simulink model "Cau_7_TDM_PCM"  (R2019a)
settings: Solver=VariableStepAuto  StartTime=0.0  StopTime=10.0  RelTol=1e-3
libraries: commutil2 x4, dspquant2 x4, dsparch4 x2, dspsigops x2, dspindex x1
settings Model: Creator=Thanh_Hai  LastModifiedBy=Thanh_Hai

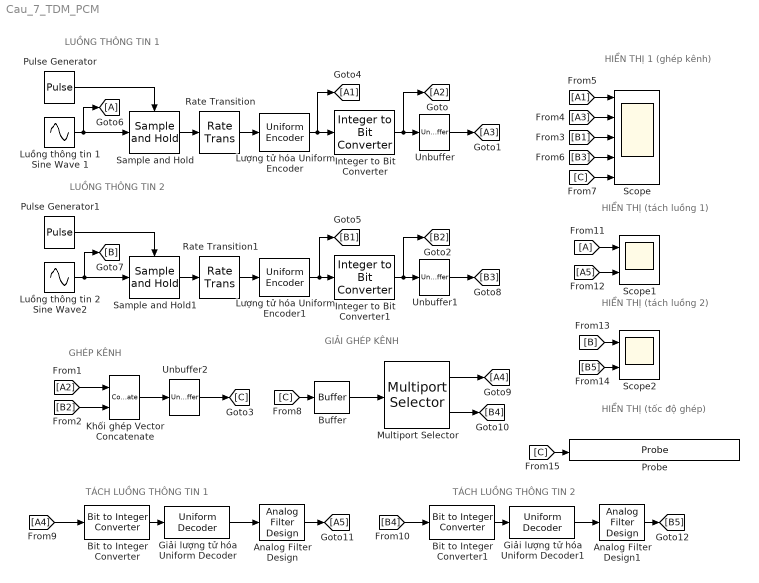
== system Cau_7_TDM_PCM ==
  note: GHÉP KÊNH
  note: LUỒNG THÔNG TIN 2
  note: HIỂN THỊ 1
      | (ghép kênh)
  note: LUỒNG THÔNG TIN 1
  note: HIỂN THỊ
      | (tách luồng 2)
  note: HIỂN THỊ
      | (tách luồng 1)
  note: GIẢI GHÉP KÊNH
  note: TÁCH LUỒNG THÔNG TIN 1
  note: TÁCH LUỒNG THÔNG TIN 2
  note: HIỂN THỊ
      | (tốc độ ghép)
  Analog Filter Design : dsparch4/Analog Filter Design  method=Butterworth  filttype=Lowpass  N=12  Wlo=2*pi*2500  Whi=80  Rp=2  Rs=40
  Analog Filter Design1 : dsparch4/Analog Filter Design  method=Butterworth  filttype=Lowpass  N=12  Wlo=2*pi*1500  Whi=80  Rp=2  Rs=40
  Bit to Integer Converter : commutil2/Bit to Integer Converter  nbits=3  bitOrder=MSB first  signedOutputValues=Unsigned  outDtype=Inherit via internal rule  outDtypeSigned=Inherit via internal rule
      settings: SourceProductName=Communications Toolbox
  Bit to Integer Converter1 : commutil2/Bit to Integer Converter  nbits=3  bitOrder=MSB first  signedOutputValues=Unsigned  outDtype=Inherit via internal rule  outDtypeSigned=Inherit via internal rule
      settings: SourceProductName=Communications Toolbox
  "Buffer " : Buffer  N=6  OutputFrames=off
  Giải lượng tử hóa Uniform Decoder : dspquant2/Uniform Decoder  peak=1  bits=3  overflowMode=Saturate  otype=Double
      settings: SourceProductName=DSP System Toolbox  SourceProductBaseCode=DS
  Giải lượng tử hóa Uniform Decoder1 : dspquant2/Uniform Decoder  peak=1  bits=3  overflowMode=Saturate  otype=Double
      settings: SourceProductName=DSP System Toolbox  SourceProductBaseCode=DS
  Integer to Bit Converter : commutil2/Integer to Bit Converter  nbits=3  signedInputValues=Unsigned  bitOrder=MSB first  outDtype=Inherit via internal rule
      settings: SourceProductName=Communications Toolbox
  Integer to Bit Converter1 : commutil2/Integer to Bit Converter  nbits=3  signedInputValues=Unsigned  bitOrder=MSB first  outDtype=Inherit via internal rule
      settings: SourceProductName=Communications Toolbox
  Khối ghép Vector Concatenate : Concatenate
  Luồng thông tin 1 Sine Wave 1 : Sin  Frequency=2*pi*2000  SampleTime=1/64000
  Luồng thông tin 2 Sine Wave2 : Sin  Frequency=2*pi*1000  SampleTime=1/64000
  Lượng tử hóa Uniform Encoder : dspquant2/Uniform Encoder  peak=1  bits=3  otype=Unsigned integer
      settings: SourceProductName=DSP System Toolbox
  Lượng tử hóa Uniform Encoder1 : dspquant2/Uniform Encoder  peak=1  bits=3  otype=Unsigned integer
      settings: SourceProductName=DSP System Toolbox
  Multiport Selector : dspindex/Multiport Selector  rowsOrCols=Rows  idxCellArray={[1 2 3],[4 5 6]}  idxErrMode=Clip Index
  "Probe " : Probe  ProbeSignalDimensions=on
  Pulse Generator : DiscretePulseGenerator  PulseType=Time based  Period=1/8000  PulseWidth=50
  Pulse Generator1 : DiscretePulseGenerator  PulseType=Time based  Period=1/8000  PulseWidth=50  PhaseDelay=1/16000
  Rate Transition : RateTransition  OutPortSampleTime=1/8000
  Rate Transition1 : RateTransition  OutPortSampleTime=1/8000
  Sample and Hold : dspsigops/Sample and Hold  trig=Rising edge  initCond=0  latchinput=off
  Sample and Hold1 : dspsigops/Sample and Hold  trig=Rising edge  initCond=0  latchinput=off
  Scope : Scope  NumInputPorts=5
  Scope1 : Scope  NumInputPorts=2
  Scope2 : Scope  NumInputPorts=2
  Unbuffer : Unbuffer
  Unbuffer1 : Unbuffer
  Unbuffer2 : Unbuffer
  wires:
  Unbuffer2/1 -> [C]
  [A1] -> Scope/1
  [A3] -> Scope/2
  Luồng thông tin 1 Sine Wave 1/1 -> [A], Sample and Hold/1
  Pulse Generator/1 -> Sample and Hold/Trigger
  Pulse Generator1/1 -> Sample and Hold1/Trigger
  Luồng thông tin 2 Sine Wave2/1 -> [B], Sample and Hold1/1
  [B1] -> Scope/3
  Sample and Hold/1 -> Rate Transition/1
  Lượng tử hóa Uniform Encoder/1 -> [A1], Integer to Bit Converter/1
  Integer to Bit Converter/1 -> [A2], Unbuffer/1
  Unbuffer/1 -> [A3]
  Lượng tử hóa Uniform Encoder1/1 -> [B1], Integer to Bit Converter1/1
  Unbuffer1/1 -> [B3]
  Sample and Hold1/1 -> Rate Transition1/1
  Integer to Bit Converter1/1 -> [B2], Unbuffer1/1
  [A2] -> Khối ghép Vector Concatenate/1
  [B2] -> Khối ghép Vector Concatenate/2
  Khối ghép Vector Concatenate/1 -> Unbuffer2/1
  Rate Transition/1 -> Lượng tử hóa Uniform Encoder/1
  Rate Transition1/1 -> Lượng tử hóa Uniform Encoder1/1
  [B3] -> Scope/4
  [C] -> Scope/5
  "Buffer "/1 -> Multiport Selector/1
  [C] -> "Buffer "/1
  Multiport Selector/1 -> [A4]
  Multiport Selector/2 -> [B4]
  Bit to Integer Converter/1 -> Giải lượng tử hóa Uniform Decoder/1
  Giải lượng tử hóa Uniform Decoder/1 -> Analog Filter Design/1
  Analog Filter Design/1 -> [A5]
  Giải lượng tử hóa Uniform Decoder1/1 -> Analog Filter Design1/1
  Bit to Integer Converter1/1 -> Giải lượng tử hóa Uniform Decoder1/1
  Analog Filter Design1/1 -> [B5]
  [A] -> Scope1/1
  [A5] -> Scope1/2
  [B] -> Scope2/1
  [B5] -> Scope2/2
  [A4] -> Bit to Integer Converter/1
  [B4] -> Bit to Integer Converter1/1
  [C] -> "Probe "/1
